simulink model "SF041A_CmplncErr"  (R2013b)
settings: Solver=FixedStepDiscrete  SolverMode=SingleTasking  StartTime=0.0  StopTime=1  FixedStep=0.002  RelTol=1e-3
libraries: NxtrAbslt x2, FixdToFloat x2, FloatToFixd x2, NxtrLim x2, LnrIntrpn x2, simulink x2
Description:
  | This function calculates the compliance error that can be used to compensate for
  | stiffness in the torque path between the motor position sensor and column axis.
settings Model: Creator=Prerit Pramod  LastModifiedBy=TZ5743
settings Model: ModifiedHistory=|
  | 001
  | Initial Release
  | P. Pramod
  | 13-August-2013
  | ICR-4236
settings SolverCC: AutoInsertRateTranBlk=on  InsertRTBMode=Always
settings DataIOCC: LimitDataPoints=off  SaveFormat=Structure  ReturnWorkspaceOutputs=on
settings OptimizationCC: BlockReduction=off  InlineParams=on  ZeroExternalMemoryAtStartup=off  ZeroInternalMemoryAtStartup=off  OptimizeModelRefInitCode=on  LifeSpan=1
settings DebuggingCC: SignalInfNanChecking=error  SignalRangeChecking=warning  UnderspecifiedInitializationDetection=Simplified  SolverPrmCheckMsg=error  InheritedTsInSrcMsg=error  DiscreteInheritContinuousMsg=error  SingleTaskRateTransMsg=error  TasksWithSamePriorityMsg=error  SigSpecEnsureSampleTimeMsg=error  CheckMatrixSingularityMsg=error  ParameterUnderflowMsg=error  ParameterPrecisionLossMsg=error  ParameterTunabilityLossMsg=error  FixptConstUnderflowMsg=warning  FixptConstOverflowMsg=warning  VectorMatrixConversionMsg=error  SignalLabelMismatchMsg=error  UnconnectedInputMsg=error  UnconnectedOutputMsg=error  UnconnectedLineMsg=error  SFcnCompatibilityMsg=error  UniqueDataStoreMsg=warning  BusObjectLabelMismatch=error  RootOutportRequireBusObject=error  AssertControl=DisableAll  ModelReferenceIOMsg=error  ModelReferenceVersionMismatchMessage=warning  ModelReferenceIOMismatchMessage=error  ModelReferenceCSMismatchMessage=warning  ModelReferenceDataLoggingMessage=error  StateNameClashWarn=warning  StrictBusMsg=ErrorOnBusTreatedAsVector  NonBusSignalsTreatedAsBus=error  SFUnexpectedBacktrackingDiag=error  SFInvalidInputDataAccessInChartInitDiag=error  SFNoUnconditionalDefaultTransitionDiag=error  SFTransitionOutsideNaturalParentDiag=error  SFUnconditionalTransitionShadowingDiag=error  SFUndirectedBroadcastEventsDiag=error
settings ModelReferenceCC: ModelReferenceNumInstancesAllowed=Single
settings RTWCC: SystemTargetFile=autosar.tlc  GenCodeOnly=on  TemplateMakefile=ert_default_tmf  Description=AUTOSAR  GenerateReport=on  ProcessScript=autosar_make_rtw_hook  LaunchReport=on
settings CodeAppCC: GenerateComments=off  IgnoreCustomStorageClasses=off  CustomSymbolStrType=$N$R$M  CustomSymbolStrBlkIO=$N$M  SimulinkBlockComments=off
settings STFCustomTargetCC: ParMdlRefBuildCompliant=on  CompOptLevelCompliant=on  IncludeMdlTerminateFcn=off  CombineOutputUpdateFcns=on  SuppressErrorStatus=on  ERTFirstTimeCompliant=on  ERTCustomFileBanners=on  SupportNonFinite=off  SupportComplex=off  SupportContinuousTime=off  SupportNonInlinedSFcns=off  MATLABClassNameForMDSCustomization=Simulink.SoftwareTarget.ERTCustomization  AutosarCompliant=on  GRTInterface=off  SystemTargetFile=autosar.tlc
settings ERTTargetCC: CodeReplacementLibrary=ANSI_C  ConcurrentExecutionCompliant=off  IncludeMdlTerminateFcn=off  SuppressErrorStatus=on  SupportNonFinite=off  SupportComplex=off  ModelStepFunctionPrototypeControlCompliant=off  CPPClassGenCompliant=off  AutosarCompliant=on  InlinedParameterPlacement=NonHierarchical  ERTCustomFileTemplate=example_file_process.tlc  EnableUserReplacementTypes=on

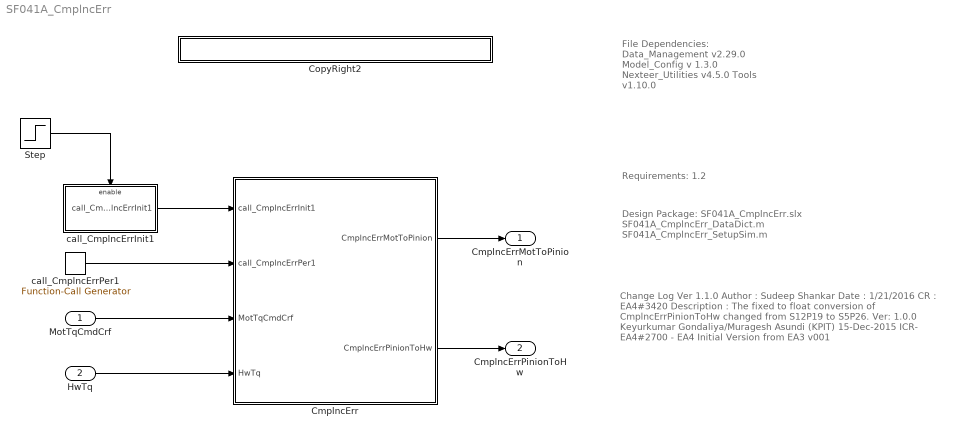
== system SF041A_CmplncErr ==
  note: Change Log
      |
      | Ver 1.1.0
      | Author : Sudeep Shankar
      | Date : 1/21/2016
      | CR : EA4#3420
      | Description : The fixed to float conversion of CmplncErrPinionToHw
      | changed from S12P19 to S5P26.
      |
      | Ver: 1.0.0
      | Keyurkumar Gondaliya/Muragesh Asundi (KPIT)
      | 15-Dec-2015
      | ICR- EA4#2700
      | - EA4 Initial Version from EA3 v001
  note: File Dependencies:
      |
      | Data_Management v2.29.0
      | Model_Config v 1.3.0
      | Nexteer_Utilities v4.5.0
      | Tools v1.10.0
  note: Design Package:
      | SF041A_CmplncErr.slx
      | SF041A_CmplncErr_DataDict.m
      | SF041A_CmplncErr_SetupSim.m
  note: Requirements: 1.2
  MotTqCmdCrf : Inport
  HwTq : Inport  Port=2
  CmplncErr : Subsystem
  CopyRight2 : Subsystem  Description=|  mask(Copyright Information){none=on}
      | Copyright info block.                                               
      |                                                                     
      | Place copyright information at the top of every subsystem in design.
      mask prompts: none "No parameters"
      mask help: Place copyright information at the top of every subsystem in design.
      mask Display:
      | NxtrConf = 'Nexteer Confidential';
      | 
      | sys = bdroot; %handle for the current model ("system")
      | first = get_param(sys,'Created');
      | first = first(end-3:end);  %year is last four digits
      | 
      | last = get_param(sys,'LastModifiedDate');
      | if isempty(last)
      |     last = datestr(now,'yyyy');
      | else
      |     last = last(end-3:end);
      | end
      | 
      | if strcmp(first,last)
      |     fprintf('%s -- Copyright %s Nexteer',NxtrConf,first)
      | else
      |     fprintf('%s -- %s%s- %s Nexteer',NxtrConf,char(169),first,last)
      | end
  Step : Step  Time=0.002  Before=1  After=0  SampleTime=0
  call_CmplncErrInit1 : Subsystem  TreatAsAtomicUnit=on
  call_CmplncErrPer1 : simulink/Ports & Subsystems/Function-Call Generator  sample_time=0.002  numberOfIterations=1
  CmplncErrMotToPinion : Outport
  CmplncErrPinionToHw : Outport  Port=2
  wires:
  CmplncErr/1(CmplncErrMotToPinion) -> CmplncErrMotToPinion/1
  CmplncErr/2(CmplncErrPinionToHw) -> CmplncErrPinionToHw/1
  Step/1 -> call_CmplncErrInit1/Enable
  call_CmplncErrInit1/1(call_CmplncErrInit1) -> CmplncErr/1(call_CmplncErrInit1)
  call_CmplncErrPer1/1 -> CmplncErr/2(call_CmplncErrPer1)
  MotTqCmdCrf/1 -> CmplncErr/3(MotTqCmdCrf)
  HwTq/1 -> CmplncErr/4(HwTq)

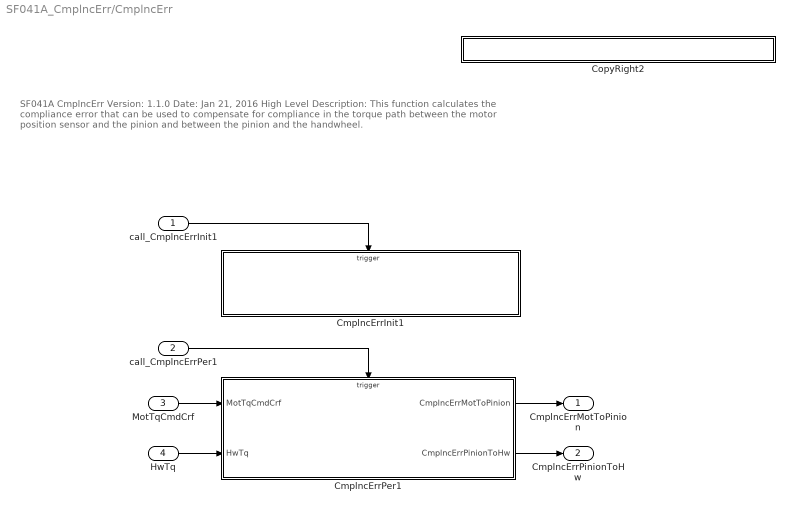
== system SF041A_CmplncErr/CmplncErr ==
  note: SF041A CmplncErr       Version: 1.1.0                                         Date:  Jan 21, 2016
      |
      | High Level Description:
      | This function calculates the compliance error that can be used to compensate
      | for compliance in the torque path between the motor position sensor and the pinion
      | and between the pinion and the handwheel.
  call_CmplncErrInit1 : Inport
  call_CmplncErrPer1 : Inport  Port=2
  MotTqCmdCrf : Inport  RequirementInfo={'linktype_rmi_doors' '0000a556 (/E-STEER Core/SubSystem Specifications/Application Functions/SF041A Compliance Error)' '#SF041A_9' 'true' 'REQ: SF041A_9' '' } %GIDa_71686f38_0272_4e5e_9658_54cb47562c1b  Port=3
  HwTq : Inport  RequirementInfo={'linktype_rmi_doors' '0000a556 (/E-STEER Core/SubSystem Specifications/Application Functions/SF041A Compliance Error)' '#SF041A_37' 'true' 'REQ: SF041A_37' '' } %GIDa_110ced84_8df1_4030_bc77_25286f5040dc  Port=4
  CmplncErrInit1 : Subsystem  TreatAsAtomicUnit=on
  CmplncErrPer1 : Subsystem  Tag=Compliance Error Calculation
      settings: AttributesFormatString=%<Tag>
  CopyRight2 : Subsystem  Description=|  mask(Copyright Information){none=on}
      | Copyright info block.                                               
      |                                                                     
      | Place copyright information at the top of every subsystem in design.
      mask prompts: none "No parameters"
      mask help: Place copyright information at the top of every subsystem in design.
      mask Display:
      | NxtrConf = 'Nexteer Confidential';
      | 
      | sys = bdroot; %handle for the current model ("system")
      | first = get_param(sys,'Created');
      | first = first(end-3:end);  %year is last four digits
      | 
      | last = get_param(sys,'LastModifiedDate');
      | if isempty(last)
      |     last = datestr(now,'yyyy');
      | else
      |     last = last(end-3:end);
      | end
      | 
      | if strcmp(first,last)
      |     fprintf('%s -- Copyright %s Nexteer',NxtrConf,first)
      | else
      |     fprintf('%s -- %s%s- %s Nexteer',NxtrConf,char(169),first,last)
      | end
  CmplncErrMotToPinion : Outport  RequirementInfo={'linktype_rmi_doors' '0000a556 (/E-STEER Core/SubSystem Specifications/Application Functions/SF041A Compliance Error)' '#SF041A_11' 'true' 'REQ: SF041A_11' '' } %GIDa_afcfc38d_9a7a_4c33_bfd1_f66d8285897e
  CmplncErrPinionToHw : Outport  RequirementInfo={'linktype_rmi_doors' '0000a556 (/E-STEER Core/SubSystem Specifications/Application Functions/SF041A Compliance Error)' '#SF041A_44' 'true' 'REQ: SF041A_44' '' } %GIDa_ad22a4ee_eb57_4902_bdbb_0fdb4d134245  Port=2
  wires:
  CmplncErrPer1/1(CmplncErrMotToPinion) -> CmplncErrMotToPinion/1
  CmplncErrPer1/2(CmplncErrPinionToHw) -> CmplncErrPinionToHw/1
  call_CmplncErrInit1/1 -> CmplncErrInit1/Trigger
  call_CmplncErrPer1/1 -> CmplncErrPer1/Trigger
  MotTqCmdCrf/1 -> CmplncErrPer1/1(MotTqCmdCrf)
  HwTq/1 -> CmplncErrPer1/2(HwTq)

== system SF041A_CmplncErr/CopyRight2 ==

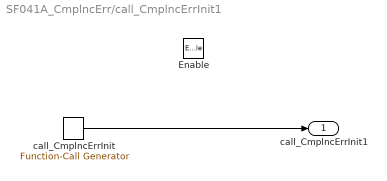
== system SF041A_CmplncErr/call_CmplncErrInit1 ==
  Enable : EnablePort
  "call_CmplncErrInit " : simulink/Ports & Subsystems/Function-Call Generator  sample_time=0  numberOfIterations=1
  call_CmplncErrInit1 : Outport
  wires:
  "call_CmplncErrInit "/1 -> call_CmplncErrInit1/1

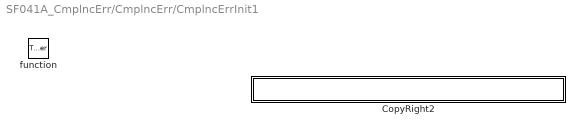
== system SF041A_CmplncErr/CmplncErr/CmplncErrInit1 ==
  function : TriggerPort  TriggerType=function-call
  CopyRight2 : Subsystem  Description=|  mask(Copyright Information){none=on}
      | Copyright info block.                                               
      |                                                                     
      | Place copyright information at the top of every subsystem in design.
      mask prompts: none "No parameters"
      mask help: Place copyright information at the top of every subsystem in design.
      mask Display:
      | NxtrConf = 'Nexteer Confidential';
      | 
      | sys = bdroot; %handle for the current model ("system")
      | first = get_param(sys,'Created');
      | first = first(end-3:end);  %year is last four digits
      | 
      | last = get_param(sys,'LastModifiedDate');
      | if isempty(last)
      |     last = datestr(now,'yyyy');
      | else
      |     last = last(end-3:end);
      | end
      | 
      | if strcmp(first,last)
      |     fprintf('%s -- Copyright %s Nexteer',NxtrConf,first)
      | else
      |     fprintf('%s -- %s%s- %s Nexteer',NxtrConf,char(169),first,last)
      | end

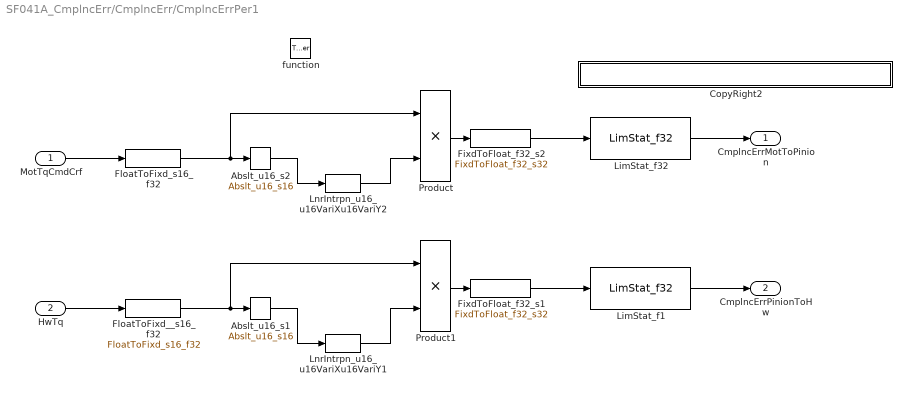
== system SF041A_CmplncErr/CmplncErr/CmplncErrPer1 ==
  MotTqCmdCrf : Inport  RequirementInfo={'linktype_rmi_doors' '0000a556 (/E-STEER Core/SubSystem Specifications/Application Functions/SF041A Compliance Error)' '#SF041A_63' 'true' 'REQ: SF041A_63' '' } %GIDa_5289f0f3_030e_4a8c_9ca6_33ef9c12f610
  HwTq : Inport  RequirementInfo={'linktype_rmi_doors' '0000a556 (/E-STEER Core/SubSystem Specifications/Application Functions/SF041A Compliance Error)' '#SF041A_65' 'true' 'REQ: SF041A_65' '' } %GIDa_6bcc2810_1377_46dd_bdce_4ad9899bc567  Port=2
  function : TriggerPort  TriggerType=function-call
  Abslt_u16_s1 : NxtrAbslt/Abslt_u16_s16  SFunctionSpec=uint16 y1 = Abslt_u16_s16( int16 u1)
      settings: AttributesFormatString=%<Name>
  Abslt_u16_s2 : NxtrAbslt/Abslt_u16_s16  SFunctionSpec=uint16 y1 = Abslt_u16_s16( int16 u1)
      settings: AttributesFormatString=%<Name>
  CopyRight2 : Subsystem  Description=|  mask(Copyright Information){none=on}
      | Copyright info block.                                               
      |                                                                     
      | Place copyright information at the top of every subsystem in design.
      mask prompts: none "No parameters"
      mask help: Place copyright information at the top of every subsystem in design.
      mask Display:
      | NxtrConf = 'Nexteer Confidential';
      | 
      | sys = bdroot; %handle for the current model ("system")
      | first = get_param(sys,'Created');
      | first = first(end-3:end);  %year is last four digits
      | 
      | last = get_param(sys,'LastModifiedDate');
      | if isempty(last)
      |     last = datestr(now,'yyyy');
      | else
      |     last = last(end-3:end);
      | end
      | 
      | if strcmp(first,last)
      |     fprintf('%s -- Copyright %s Nexteer',NxtrConf,first)
      | else
      |     fprintf('%s -- %s%s- %s Nexteer',NxtrConf,char(169),first,last)
      | end
  FixdToFloat_f32_s1 : FixdToFloat/FixdToFloat_f32_s32  Param1=26
  FixdToFloat_f32_s2 : FixdToFloat/FixdToFloat_f32_s32  Param1=19
  FloatToFixd__s16_f32 : FloatToFixd/FloatToFixd_s16_f32  Param1=11
  FloatToFixd_s16_f32 : FloatToFixd/FloatToFixd_s16_f32  Param1=11
  LimStat_f1 : NxtrLim/LimStat_f32  RequirementInfo={'linktype_rmi_doors' '0000a556 (/E-STEER Core/SubSystem Specifications/Application Functions/SF041A Compliance Error)' '#SF041A_66' 'true' 'REQ: SF041A_66' '' ; 'linktype_rmi_doors' '0000a556 (/E-STEER Core/SubSystem Specifications/Application Functions/SF041A Compliance Error)' '#SF041A_51' 'true' 'REQ: SF041A_51' '' ; 'linktype_rmi_doors' '0000a556 (/E-STEER Core/SubSystem Specifications/Application Functions/SF041A Compliance Error)' '#SF041A_42' 'true' 'REQ: SF041A_42' '' } %GIDa_4c905fb3_6594_4ecc_86b2_6568c88ff519  LoLim=CMPLNCERRPINIONTOHWMIN_HWDEG_F32  HiLim=CMPLNCERRPINIONTOHWMAX_HWDEG_F32
      settings: AttributesFormatString=|
      | Low Limit: %<LoLim>
      | High Limit:%<HiLim>
  LimStat_f32 : NxtrLim/LimStat_f32  RequirementInfo={'linktype_rmi_doors' '0000a556 (/E-STEER Core/SubSystem Specifications/Application Functions/SF041A Compliance Error)' '#SF041A_64' 'true' 'REQ: SF041A_64' '' ; 'linktype_rmi_doors' '0000a556 (/E-STEER Core/SubSystem Specifications/Application Functions/SF041A Compliance Error)' '#SF041A_52' 'true' 'REQ: SF041A_52' '' ; 'linktype_rmi_doors' '0000a556 (/E-STEER Core/SubSystem Specifications/Application Functions/SF041A Compliance Error)' '#SF041A_42' 'true' 'REQ: SF041A_42' '' } %GIDa_7d2e5f8c_04ca_49a2_a910_2897c0efb13f  LoLim=CMPLNCERRMOTTOPINIONMIN_HWDEG_F32  HiLim=CMPLNCERRMOTTOPINIONMAX_HWDEG_F32
      settings: AttributesFormatString=|
      | Low Limit: %<LoLim>
      | High Limit:%<HiLim>
  LnrIntrpn_u16_u16VariXu16VariY1 : LnrIntrpn/LnrIntrpn_u16_u16VariXu16VariY  RequirementInfo={'linktype_rmi_doors' '0000a556 (/E-STEER Core/SubSystem Specifications/Application Functions/SF041A Compliance Error)' '#SF041A_62' 'true' 'REQ: SF041A_62' '' ; 'linktype_rmi_doors' '0000a556 (/E-STEER Core/SubSystem Specifications/Application Functions/SF041A Compliance Error)' '#SF041A_49' 'true' 'REQ: SF041A_49' '' ; 'linktype_rmi_doors' '0000a556 (/E-STEER Core/SubSystem Specifications/Application Functions/SF041A Compliance Error)' '#SF041A_53' 'true' 'REQ: SF041A_53' '' } %GIDa_95cf2954_41d3_4910_ba5a_dcbfa53bc342  XTbl=CmplncErrHwAgNonLinCmplncIndTblX  YTbl=CmplncErrHwAgNonLinCmplncDepTblY
      settings: AttributesFormatString=Lnr ( u16VariX , u16VariY )
  LnrIntrpn_u16_u16VariXu16VariY2 : LnrIntrpn/LnrIntrpn_u16_u16VariXu16VariY  RequirementInfo={'linktype_rmi_doors' '0000a556 (/E-STEER Core/SubSystem Specifications/Application Functions/SF041A Compliance Error)' '#SF041A_36' 'true' 'REQ: SF041A_36' '' ; 'linktype_rmi_doors' '0000a556 (/E-STEER Core/SubSystem Specifications/Application Functions/SF041A Compliance Error)' '#SF041A_40' 'true' 'REQ: SF041A_40' '' ; 'linktype_rmi_doors' '0000a556 (/E-STEER Core/SubSystem Specifications/Application Functions/SF041A Compliance Error)' '#SF041A_54' 'true' 'REQ: SF041A_54' '' ; 'linktype_rmi_doors' '0000a556 (/E-STEER Core/SubSystem Specifications/Application Functions/SF041A Compliance Error)' '#SF041A_56' 'true' 'REQ: SF041A_56' '' ; 'linktype_rmi_doors' '0000a556 (/E-STEER Core/SubSystem Specifications/Application Functions/SF041A Compliance Error)' '#SF041A_57' 'true' 'REQ: SF041A_57' '' } %GIDa_1109f467_3ade_4ef0_83bb_0e5b662857b7  XTbl=CmplncErrMotAgNonLinCmplncIndTblX  YTbl=CmplncErrMotAgNonLinCmplncDepTblY
      settings: AttributesFormatString=Lnr ( u16VariX , u16VariY )
  Product : Product  RequirementInfo={'linktype_rmi_doors' '0000a556 (/E-STEER Core/SubSystem Specifications/Application Functions/SF041A Compliance Error)' '#SF041A_35' 'true' 'REQ: SF041A_35' '' } %GIDa_010d08a8_c170_4733_bfb9_51b9c8fc004a  RndMeth=Zero
  Product1 : Product  RequirementInfo={'linktype_rmi_doors' '0000a556 (/E-STEER Core/SubSystem Specifications/Application Functions/SF041A Compliance Error)' '#SF041A_38' 'true' 'REQ: SF041A_38' '' } %GIDa_54613647_0770_46ca_b2f9_ab91932acd68  RndMeth=Zero
  CmplncErrMotToPinion : Outport  RequirementInfo={'linktype_rmi_doors' '0000a556 (/E-STEER Core/SubSystem Specifications/Application Functions/SF041A Compliance Error)' '#SF041A_47' 'true' 'REQ: SF041A_47' '' ; 'linktype_rmi_doors' '0000a556 (/E-STEER Core/SubSystem Specifications/Application Functions/SF041A Compliance Error)' '#SF041A_39' 'true' 'REQ: SF041A_39' '' ; 'linktype_rmi_doors' '0000a556 (/E-STEER Core/SubSystem Specifications/Application Functions/SF041A Compliance Error)' '#SF041A_41' 'true' 'REQ: SF041A_41' '' } %GIDa_3db6d88b_a924_4929_8aef_93b68b960585
  CmplncErrPinionToHw : Outport  RequirementInfo={'linktype_rmi_doors' '0000a556 (/E-STEER Core/SubSystem Specifications/Application Functions/SF041A Compliance Error)' '#SF041A_48' 'true' 'REQ: SF041A_48' '' ; 'linktype_rmi_doors' '0000a556 (/E-STEER Core/SubSystem Specifications/Application Functions/SF041A Compliance Error)' '#SF041A_39' 'true' 'REQ: SF041A_39' '' ; 'linktype_rmi_doors' '0000a556 (/E-STEER Core/SubSystem Specifications/Application Functions/SF041A Compliance Error)' '#SF041A_41' 'true' 'REQ: SF041A_41' '' } %GIDa_7179793d_0c2f_44c3_ab37_f80db9334464  Port=2
  wires:
  MotTqCmdCrf/1 -> FloatToFixd_s16_f32/1
  Abslt_u16_s2/1 -> LnrIntrpn_u16_u16VariXu16VariY2/1
  FloatToFixd_s16_f32/1 -> Abslt_u16_s2/1, Product/1
  Product/1 -> FixdToFloat_f32_s2/1
  FixdToFloat_f32_s2/1 -> LimStat_f32/1
  FixdToFloat_f32_s1/1 -> LimStat_f1/1
  Product1/1 -> FixdToFloat_f32_s1/1
  HwTq/1 -> FloatToFixd__s16_f32/1
  FloatToFixd__s16_f32/1 -> Abslt_u16_s1/1, Product1/1
  Abslt_u16_s1/1 -> LnrIntrpn_u16_u16VariXu16VariY1/1
  LnrIntrpn_u16_u16VariXu16VariY2/1 -> Product/2
  LnrIntrpn_u16_u16VariXu16VariY1/1 -> Product1/2
  LimStat_f32/1 -> CmplncErrMotToPinion/1
  LimStat_f1/1 -> CmplncErrPinionToHw/1

== system SF041A_CmplncErr/CmplncErr/CopyRight2 ==

== system SF041A_CmplncErr/CmplncErr/CmplncErrInit1/CopyRight2 ==

== system SF041A_CmplncErr/CmplncErr/CmplncErrPer1/CopyRight2 ==
